simulink library "Mako_Dynamics"  (R2024b)
settings: Solver=VariableStepAuto  StartTime=0.0  StopTime=10.0  RelTol=1e-3
settings Model: Creator=pinto  LastModifiedBy=pinto

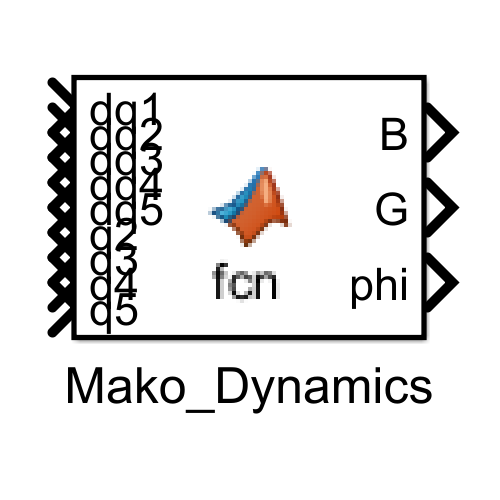
[thumbnail: Simulink's stored preview of the top-level diagram]
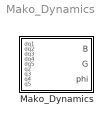
== system Mako_Dynamics ==
  Mako_Dynamics : MATLAB Function  TreatAsAtomicUnit=on

== matlab function Mako_Dynamics/Mako_Dynamics ==
  data: dq1 input; B output; dq2 input; dq3 input; dq4 input; dq5 input; q2 input; q3 input; q4 input; q5 input; G output; phi output
function [B,G,phi] = Mako_Dynamics(dq1,dq2,dq3,dq4,dq5,q2,q3,q4,q5)
%#codegen

%    This function was generated by the Symbolic Math Toolbox version 24.2.
%    17-Jun-2025 19:39:53

% dq1 = complex(dq1);  % if required to enforce complex operations
% dq2 = complex(dq2);  % if required to enforce complex operations
% dq3 = complex(dq3);  % if required to enforce complex operations
% dq4 = complex(dq4);  % if required to enforce complex operations
% dq5 = complex(dq5);  % if required to enforce complex operations
% q2 = complex(q2);  % if required to enforce complex operations
% q3 = complex(q3);  % if required to enforce complex operations
% q4 = complex(q4);  % if required to enforce complex operations
% q5 = complex(q5);  % if required to enforce complex operations
t2 = cos(q5);
t3 = sin(q5);
t4 = dq2.*dq3;
t7 = -dq5;
t8 = pi./2.0;
t17 = dq4.*6.66539706722529e-3;
t113 = dq5.*5.289063987811844e-2;
t114 = dq3.*6.155821510188537e-2;
t5 = t2.^2;
t6 = t3.^2;
t9 = -t8;
t10 = q2+t8;
t11 = q3+t8;
t117 = -t113;
t12 = q4+t9;
t13 = cos(t10);
t14 = cos(t11);
t15 = sin(t10);
t16 = sin(t11);
t120 = t6.*5.289063987811844e-2;
t121 = t5.*9.371072176728241e-3;
t18 = cos(t12);
t19 = sin(t12);
t20 = dq1.*t13;
t21 = dq2.*t14;
t22 = dq2.*t16;
t24 = dq1.*dq2.*t15;
t27 = t16.*(2.0./5.0);
t44 = t16.*4.570557988954485e-1;
t45 = dq1.*t14.*t15;
t46 = dq1.*t15.*t16;
t49 = t14.*t15.*(2.0./5.0);
t70 = t14.*t15.*4.570557988954485e-1;
t75 = t15.*t16.*1.120929346791087e+1;
t80 = t14.*t15.*5.254356313083222;
t81 = t15.*t16.*9.738073700247572;
t92 = t2.*t15.*t16.*2.269881927251952e+1;
t93 = t3.*t15.*t16.*2.269881927251952e+1;
t131 = t2.*t14.*9.371072176728241e-3;
t132 = t3.*t14.*5.289063987811844e-2;
t153 = t14.*1.149037088173681e-1;
t154 = t16.*3.247223743096553e-1;
t160 = t2.*t15.*t16.*9.371072176728241e-3;
t163 = t3.*t15.*t16.*5.289063987811844e-2;
t191 = t14.*t15.*3.247223743096553e-1;
t192 = t15.*t16.*1.149037088173681e-1;
t23 = dq2.*t20;
t25 = t18.^2;
t26 = t19.^2;
t28 = dq3+t20;
t31 = t21./4.0;
t32 = t21.*(2.0./5.0);
t33 = t22./4.0;
t34 = t22.*(2.0./5.0);
t39 = t19.*6.66539706722529e-3;
t41 = t21.*6.66539706722529e-3;
t42 = t13.*t18;
t43 = t13.*t19;
t47 = dq3.*t46;
t48 = dq3.*t45;
t50 = -t45;
t51 = t45./4.0;
t52 = t45.*(2.0./5.0);
t54 = t46./4.0;
t55 = dq1.*t15.*t27;
t65 = t16.*t18.*6.66539706722529e-3;
t66 = t46.*6.66539706722529e-3;
t67 = t14.*t15.*t18;
t68 = t14.*t15.*t19;
t73 = t14.*t18.*4.570557988954485e-1;
t74 = t14.*t19.*1.382593791658732;
t76 = dq1.*dq3.*t15.*t44;
t79 = t3.*t14.*t18.*9.255379927632832e-1;
t83 = t21+t46;
t87 = t2.*t14.*t18.*9.255379927632832e-1;
t104 = t15.*t18.*t44;
t105 = t15.*t16.*t19.*1.382593791658732;
t112 = t3.*t15.*t16.*t18.*9.255379927632832e-1;
t115 = t2.*t15.*t16.*t18.*9.255379927632832e-1;
t126 = t21.*2.789647210055228e-2;
t127 = t20.*6.155821510188537e-2;
t128 = t22.*6.155821510188537e-2;
t130 = t18.*5.289063987811844e-2;
t140 = t5.*t19.*5.289063987811844e-2;
t142 = t6.*t19.*9.371072176728241e-3;
t145 = t2.*t3.*t19.*4.35195677013902e-2;
t147 = t18.*5.860383736431155e-2;
t152 = t46.*2.789647210055228e-2;
t155 = t45.*6.155821510188537e-2;
t157 = t16.*t19.*5.289063987811844e-2;
t166 = t3.*t16.*t18.*9.371072176728241e-3;
t171 = t2.*t16.*t18.*(-5.289063987811844e-2);
t185 = t16.*t19.*5.860383736431155e-2;
t29 = -t23;
t35 = dq4.*t28;
t37 = t25./1.0e+1;
t38 = t26./1.0e+1;
t53 = t25.*3.456484479146829e-1;
t56 = t26.*3.456484479146829e-1;
t58 = dq3.*t55;
t59 = -t51;
t60 = -t52;
t61 = t18.*t28;
t62 = t19.*t28;
t63 = t48.*(2.0./5.0);
t64 = t13.*t39;
t69 = t43.*(9.81e+2./1.0e+2);
t77 = -t68;
t78 = t43.*1.120929346791087e+1;
t84 = t28.*t39;
t89 = dq4+t83;
t90 = t42.*3.390811274043039e+1;
t94 = t22+t50;
t98 = t67.*6.66539706722529e-3;
t103 = t67.*(9.81e+2./1.0e+2);
t106 = t31+t54;
t107 = t32+t55;
t109 = t67.*1.120929346791087e+1;
t116 = t68.*3.390811274043039e+1;
t129 = t43+t67;
t133 = -t130;
t148 = t17+t41+t66;
t156 = t42.*5.289063987811844e-2;
t161 = -t155;
t164 = -t157;
t184 = t42.*5.860383736431155e-2;
t194 = t68.*5.289063987811844e-2;
t199 = t47.*3.247223743096553e-1;
t200 = t48.*1.149037088173681e-1;
t210 = t68.*5.860383736431155e-2;
t242 = t114+t127;
t251 = t126+t152;
t256 = t131+t166;
t259 = t132+t171;
t307 = t39+t140+t142;
t36 = -t35;
t40 = t4+t29;
t82 = t61.*5.713197486193106e-3;
t96 = t89.^2;
t97 = dq5.*t89;
t99 = t2.*t89;
t100 = t3.*t89;
t101 = dq4.*t94;
t102 = t37+t38;
t110 = t33+t59;
t111 = t34+t60;
t119 = -t116;
t122 = t19.*t94;
t123 = t18.*t94;
t124 = t53+t56;
t134 = t42+t77;
t138 = t28.*t107;
t162 = -t156;
t177 = t61.*5.289063987811844e-2;
t180 = t28.*t106.*5.356122643306037e-1;
t193 = t69+t103;
t203 = t83.*t107;
t216 = -t210;
t241 = t2.*t129.*5.289063987811844e-2;
t243 = t3.*t129.*9.371072176728241e-3;
t253 = t128+t161;
t265 = t2.*t256;
t266 = t3.*t256;
t267 = t2.*t259;
t268 = t3.*t259;
t287 = t28.*t251;
t294 = t83.*t242;
t303 = t94.*t242;
t315 = t18.*t307;
t316 = t19.*t307;
t321 = t94.*t251;
t71 = t14.*t40;
t72 = t16.*t40;
t125 = -t123;
t136 = t122.*5.713197486193106e-3;
t139 = t123.*6.66539706722529e-3;
t141 = t28.*t111;
t144 = -t138;
t146 = t16.*t19.*t102;
t149 = t18.*t102.*4.570557988954485e-1;
t150 = t18.*t102.*1.142639497238621;
t151 = t14.*t102.*3.456484479146829;
t168 = t19.*t124.*(2.0./5.0);
t169 = t5.*t18.*t102.*9.255379927632832e-1;
t170 = t6.*t18.*t102.*9.255379927632832e-1;
t173 = t5.*t18.*t102.*2.313844981908208;
t175 = t6.*t18.*t102.*2.313844981908208;
t178 = t138.*1.142639497238621;
t181 = t28.*t110.*5.356122643306037e-1;
t183 = t138.*9.926680632260522e-1;
t190 = t15.*t16.*t102.*3.456484479146829;
t201 = t61+t122;
t206 = t96.*t102;
t208 = t100.*5.289063987811844e-2;
t209 = t99.*9.371072176728241e-3;
t212 = t94.*t111;
t218 = t90+t119;
t226 = t2.*t193.*2.313844981908208;
t227 = t3.*t193.*2.313844981908208;
t230 = t122.*5.289063987811844e-2;
t231 = t102.*t124;
t239 = t102.*t134;
t271 = -t267;
t290 = t28.*t253;
t295 = -t287;
t304 = t162+t194;
t309 = -t303;
t319 = t83.*t253;
t325 = t163+t241;
t332 = -t3.*(t160-t243);
t335 = t2.*(t160-t243);
t85 = t71.*(2.0./5.0);
t91 = t72.*(-2.0./5.0);
t108 = t71.*4.570557988954485e-1;
t143 = -t139;
t158 = -t151;
t159 = -t146;
t172 = -t168;
t179 = -t178;
t182 = t141.*5.356122643306037e-1;
t186 = -t181;
t187 = -t183;
t189 = t146.*1.142639497238621;
t195 = t146.*(-4.570557988954485e-1);
t197 = -t190;
t198 = t36+t47+t71;
t204 = t62+t125;
t205 = t201.^2;
t214 = t7+t201;
t219 = t71.*3.247223743096553e-1;
t220 = t72.*1.149037088173681e-1;
t228 = t206.*1.142639497238621;
t232 = t82+t136;
t240 = t19.*t218.*(2.0./5.0);
t245 = t239.*4.570557988954485e-1;
t246 = t239.*1.142639497238621;
t254 = t49+t239;
t261 = t102.*t218;
t269 = t93+t226;
t281 = -t3.*(t92-t227);
t288 = t2.*(t92-t227);
t310 = t148.*t201;
t322 = -t319;
t324 = t203+t212;
t329 = t2.*t325;
t330 = t3.*t325;
t356 = t150+t173+t175;
t357 = t117+t177+t230;
t370 = t65+t266+t271;
t196 = -t189;
t207 = t27+t159;
t213 = dq5.*t204;
t215 = t2.*t204;
t217 = t3.*t204;
t222 = -t220;
t223 = t18.*t198;
t224 = t19.*t198;
t233 = t84+t143;
t238 = t74+t158;
t244 = -t240;
t249 = t105+t197;
t252 = t102.*t205;
t257 = t63+t91+t141;
t274 = t89.*t232;
t275 = t2.*t269;
t276 = t3.*t269;
t296 = t288.*(2.0./5.0);
t298 = t2.*t254.*2.313844981908208;
t301 = t3.*t254.*2.313844981908208;
t311 = t148.*t204;
t317 = t89.*t102.*t204;
t333 = t19.*t324;
t336 = t204.*t232;
t341 = t18.*t324.*3.456484479146829;
t362 = t102.*t201.*t204.*3.456484479146829;
t366 = t102.*t356;
t369 = t120+t121+t172+t231+6.66539706722529e-3;
t373 = t18.*t370;
t374 = t19.*t370;
t397 = t64+t98+t329+t332;
t221 = -t217;
t234 = t223.*6.66539706722529e-3;
t235 = t2.*t207.*2.313844981908208;
t236 = t3.*t207.*2.313844981908208;
t248 = t19.*t238.*(2.0./5.0);
t258 = t100+t215;
t260 = t217.*9.371072176728241e-3;
t262 = t215.*5.289063987811844e-2;
t273 = t252.*1.142639497238621;
t279 = t89.*t233;
t282 = t19.*t249.*(2.0./5.0);
t284 = t18.*t257;
t289 = t276.*(2.0./5.0);
t297 = t224.*5.860383736431155e-2;
t302 = t102.*t238;
t314 = t19.*t257.*3.456484479146829;
t320 = t102.*t249;
t326 = t317.*4.570557988954485e-1;
t327 = t317.*1.142639497238621;
t334 = t201.*t233;
t338 = t333.*1.142639497238621;
t339 = t112+t298;
t340 = t3.*(-t48+t72+t213).*5.289063987811844e-2;
t342 = t2.*(-t48+t72+t213).*9.371072176728241e-3;
t349 = -t3.*(t115-t301);
t350 = t2.*(t115-t301);
t352 = t3.*(t115-t301).*(-2.0./5.0);
t354 = t102.*(t224-t18.*(t24-t101));
t368 = t3.*(-t97+t223+t19.*(t24-t101)).*(-9.371072176728241e-3);
t375 = t75+t276+t288;
t376 = -t374;
t377 = t147+t366;
t390 = t78+t109+t275+t281;
t399 = t18.*t397;
t400 = t19.*t397;
t263 = t99+t221;
t264 = -t260;
t272 = t87+t236;
t291 = -t2.*(t79-t235);
t299 = t3.*(t79-t235);
t306 = t2.*(t79-t235).*(-2.0./5.0);
t308 = -t302;
t312 = t284.*1.142639497238621;
t323 = -t320;
t337 = -t334;
t346 = t2.*t339;
t347 = t3.*t339;
t355 = -t354;
t358 = t208+t262;
t359 = t354.*4.570557988954485e-1;
t360 = t354.*1.142639497238621;
t379 = t18.*t377;
t380 = t19.*t377;
t383 = t258.*t357;
t391 = t19.*t102.*t375;
t393 = t18.*t390.*(2.0./5.0);
t411 = t2.*(t206+t252-t284-t333).*(-2.313844981908208);
t413 = t3.*(t206+t252-t284-t333).*2.313844981908208;
t419 = t19.*(-t314+t341+t362+t102.*(t48-t72).*3.456484479146829).*(-2.0./5.0);
t421 = t102.*(-t314+t341+t362+t102.*(t48-t72).*3.456484479146829);
t285 = t2.*t272;
t286 = t3.*t272;
t351 = t346.*(2.0./5.0);
t361 = t209+t264;
t363 = -t359;
t364 = -t360;
t371 = t214.*t358;
t381 = -t380;
t384 = t263.*t357;
t385 = -t383;
t387 = t263.*t358;
t392 = -t391;
t398 = t104+t347+t350;
t402 = t58+t85+t144+t317+t355;
t408 = t316+t379+6.155821510188537e-2;
t410 = t70+t246+t346+t349;
t415 = t80+t244+t261+t393;
t300 = t286.*(2.0./5.0);
t372 = t214.*t361;
t378 = t73+t285+t299;
t386 = t258.*t361;
t394 = t44+t196+t286+t291;
t401 = t18.*t398.*(2.0./5.0);
t404 = t2.*t402.*2.313844981908208;
t405 = t3.*t402.*2.313844981908208;
t414 = t102.*t410;
t417 = t81+t289+t296+t392;
t418 = t149+t169+t170+t315+t381;
t437 = t342+t368+t371+t385;
t382 = t18.*t378.*(2.0./5.0);
t395 = t102.*t394;
t422 = t184+t216+t414;
t428 = t405+t411;
t429 = t404+t413;
t438 = t2.*t437;
t439 = t3.*t437;
t443 = -t3.*(t340-t372+t384+t2.*(-t97+t223+t19.*(t24-t101)).*5.289063987811844e-2);
t444 = t192+t282+t323+t330+t335+t401;
t396 = -t395;
t423 = t18.*t422;
t424 = t19.*t422;
t427 = t153+t248+t265+t268+t308+t382;
t430 = t2.*t428;
t431 = t3.*t428;
t432 = t2.*t429;
t433 = t3.*t429;
t441 = -t438;
t449 = -t19.*(t234+t274-t310-t439+t39.*(t24-t101)+t2.*(t340-t372+t384+t2.*(-t97+t223+t19.*(t24-t101)).*5.289063987811844e-2));
t450 = t18.*(t234+t274-t310-t439+t39.*(t24-t101)+t2.*(t340-t372+t384+t2.*(-t97+t223+t19.*(t24-t101)).*5.289063987811844e-2));
t403 = t185+t396;
t425 = -t424;
t435 = t431.*(2.0./5.0);
t436 = t432.*(2.0./5.0);
t451 = t75+t76+t108+t179+t327+t364+t431+t432;
t453 = t18.*(t228+t273-t312-t338-t430+t433).*(-2.0./5.0);
t406 = t18.*t403;
t407 = t19.*t403;
t446 = t191+t245+t351+t352+t399+t425;
t454 = t102.*t451;
t459 = t80+t182+t186+t200+t222+t290+t309+t336+t337+t419+t421+t441+t443+t453;
t426 = t376+t406;
t445 = t154+t195+t300+t306+t373+t407;
mt1 = [t15.*(t15.*6.09407731860598e-2+t14.*t446+t16.*t444)+t13.*(t13.*1.529693748809751e-1+t400+t423)+6.509176823462196e-1,t14.*t444-t16.*t446,t13.*6.155821510188537e-2+t400+t423,t323+t330+t335+t15.*t16.*6.66539706722529e-3,t304,-t13.*(t374-t406)+t15.*(t16.*t427-t14.*t445)];
mt2 = [t14.*t427+t16.*t445+6.09407731860598e-2,t426,t14.*6.66539706722529e-3+t265+t268+t308,t164,t13.*t408+t15.*(t16.*t145+t14.*t418),t14.*t145-t16.*t418,t408,t145,t133,t15.*(t16.*t369+t2.*t3.*t14.*t18.*4.35195677013902e-2)+t2.*t3.*t43.*4.35195677013902e-2,t14.*t369-t2.*t3.*t16.*t18.*4.35195677013902e-2,t145];
mt3 = [t120+t121+t231+6.66539706722529e-3,0.0,t304,t164,t133,0.0,5.289063987811844e-2];
B = reshape([mt1,mt2,mt3],5,5);
if nargout > 1
    G = [-t15.*(t14.*t417-t16.*t415)-t42.*t102.*t375;t14.*t415+t16.*t417;-t18.*t102.*t375;t261;0.0];
end
if nargout > 2
    t457 = -t18.*(-t279-t297+t311+t386-t387+t454+t147.*(t24-t101));
    t458 = -t19.*(-t279-t297+t311+t386-t387+t454+t147.*(t24-t101));
    t460 = t81+t180+t187+t199+t219+t294+t295+t326+t363+t435+t436+t450+t458;
    mt4 = [t15.*(t23.*3.04703865930299e-2-t14.*t460+t16.*t459)-t13.*(t24.*1.529693748809751e-1+t319-t321+t18.*(-t279-t297+t311+t386-t387+t454+t147.*(t24-t101))+t19.*(t234+t274-t310-t439+t39.*(t24-t101)+t2.*(t340-t372+t384+t2.*(-t97+t223+t19.*(t24-t101)).*5.289063987811844e-2)))];
    mt5 = [t14.*t459+t16.*t460+dq1.*t15.*t20.*3.04703865930299e-2;t24.*(-6.155821510188537e-2)+t321+t322+t449+t457;t48.*6.66539706722529e-3-t72.*6.66539706722529e-3+t336+t337+t421+t441+t443;t224.*(-5.289063987811844e-2)+t386-t387+t130.*(t24-t101)];
    phi = [mt4;mt5];
end
end
